simulink library "lib_Radiation_HeatXCoeffRefConcCyl"  (R2015a)
settings: Solver=ode45  StartTime=0.0  StopTime=10.0  RelTol=1e-3
settings Model: Creator=jlkratz  LastModifiedBy=jlkratz

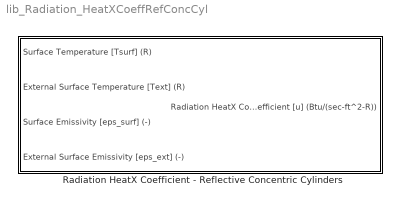
== system lib_Radiation_HeatXCoeffRefConcCyl ==
  Radiation HeatX Coefficient - Reflective Concentric Cylinders : Subsystem  mask(TSAT: Radiation HeatX Coefficient - Non-Reflective Sink Block){Rsurf_M=[0.25 0.25; 0.25 0.25];, Rext_M=[0.4 0.4; 0.4 0.4];}
      mask prompts: Rsurf_M "Rsurf_M - Radius of the surface of interest [Rsurf] (ft)"; Rext_M "Rext_M - Radius of the external surface [Rext] (ft)"
      mask help:
      | This function computes the radiation heat transfer coefficient when the radiation term is written in a linear form (q = u*(Text - Tsurf)). This block is applicable for radiation between two reflective concentric cylinder surfaces.
      |
      | Units are specified on the inport and outports so be sure to adhere to the appropriate units.
      mask Help: web(which('Radiation_TSAT_HeatXCoeffRefConcCyl.html'),'-helpbrowser')

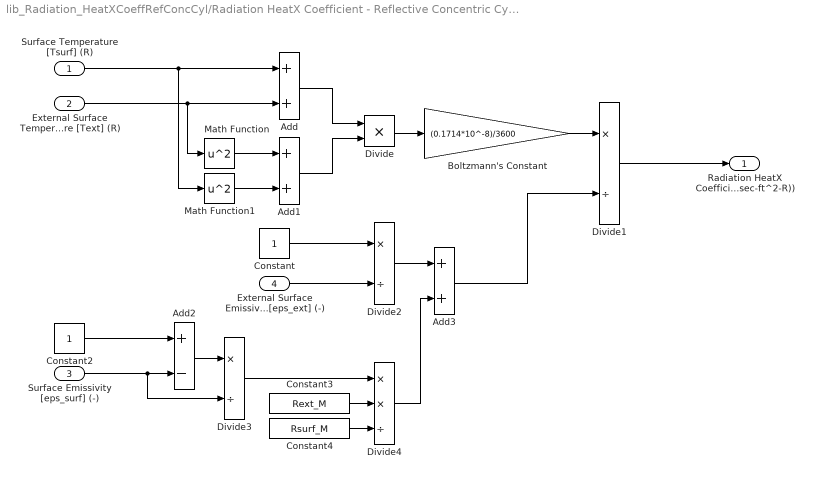
== system lib_Radiation_HeatXCoeffRefConcCyl/Radiation HeatX Coefficient - Reflective Concentric Cylinders ==
  Surface Temperature [Tsurf] (R) : Inport
  External Surface Temperature [Text] (R) : Inport  Port=2
  Surface Emissivity [eps_surf] (-) : Inport  Port=3
  External Surface Emissivity [eps_ext] (-) : Inport  Port=4
  Add : Sum
  Add1 : Sum
  Add2 : Sum  Inputs=+-
  Add3 : Sum
  Boltzmann's Constant : Gain  Gain=(0.1714*10^-8)/3600
  Constant : Constant
  Constant2 : Constant
  Constant3 : Constant  Value=Rext_M
  Constant4 : Constant  Value=Rsurf_M
  Divide : Product  Inputs=**
  Divide1 : Product  Inputs=*/
  Divide2 : Product  Inputs=*/
  Divide3 : Product  Inputs=*/
  Divide4 : Product  Inputs=**/
  Math Function : Math  Operator=square  SaturateOnIntegerOverflow=on
  Math Function1 : Math  Operator=square  SaturateOnIntegerOverflow=on
  Radiation HeatX Coefficient [u] (Btu/(sec-ft^2-R)) : Outport
  wires:
  Add3/1 -> Divide1/2
  Add2/1 -> Divide3/1
  Surface Emissivity [eps_surf] (-)/1 -> Add2/2, Divide3/2
  External Surface Emissivity [eps_ext] (-)/1 -> Divide2/2
  Divide4/1 -> Add3/2
  Constant4/1 -> Divide4/3
  Constant3/1 -> Divide4/2
  Constant2/1 -> Add2/1
  Divide3/1 -> Divide4/1
  Divide2/1 -> Add3/1
  Constant/1 -> Divide2/1
  Math Function1/1 -> Add1/2
  Divide1/1 -> Radiation HeatX Coefficient [u] (Btu/(sec-ft^2-R))/1
  Surface Temperature [Tsurf] (R)/1 -> Add/1, Math Function1/1
  External Surface Temperature [Text] (R)/1 -> Add/2, Math Function/1
  Divide/1 -> Boltzmann's Constant/1
  Add1/1 -> Divide/2
  Boltzmann's Constant/1 -> Divide1/1
  Add/1 -> Divide/1
  Math Function/1 -> Add1/1
